simulink model "Bioreactor2_fuzzy_control"  (R2016a)
settings: Solver=VariableStepAuto  StartTime=0.0  StopTime=500  RelTol=1e-3
undefined symbols (not defined in the file or in its folder): Bioreactor2FuzzyMadani, Bioreactor2FuzzySugeno, evalfis
settings Model: Creator=Daniel  LastModifiedBy=Daniel

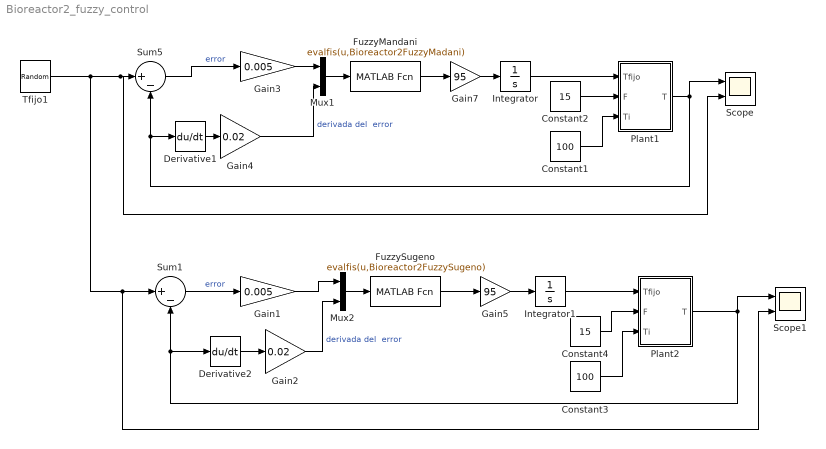
== system Bioreactor2_fuzzy_control ==
  Constant1 : Constant  Value=100
  Constant2 : Constant  Value=15
  Constant3 : Constant  Value=100
  Constant4 : Constant  Value=15
  Derivative1 : Derivative
  Derivative2 : Derivative
  FuzzyMandani : MATLABFcn  MATLABFcn=evalfis(u,Bioreactor2FuzzyMadani)  OutputDimensions=1
  FuzzySugeno : MATLABFcn  MATLABFcn=evalfis(u,Bioreactor2FuzzySugeno)  OutputDimensions=1
  Gain1 : Gain  Gain=0.005
  Gain2 : Gain  Gain=0.02
  Gain3 : Gain  Gain=0.005
  Gain4 : Gain  Gain=0.02
  Gain5 : Gain  Gain=95
  Gain7 : Gain  Gain=95
  Integrator : Integrator
  Integrator1 : Integrator
  Mux1 : Mux  Inputs=2
  Mux2 : Mux  Inputs=2
  Plant1 : Subsystem
  Plant2 : Subsystem
  Scope : Scope  NumInputPorts=2
  Scope1 : Scope  NumInputPorts=2
  Sum1 : Sum  Inputs=|+-
  Sum5 : Sum  Inputs=|+-
  Tfijo1 : UniformRandomNumber  Minimum=130  Maximum=170  SampleTime=50
  wires:
  Sum5/1 -> Gain3/1  "error"
  Gain3/1 -> Mux1/1
  Derivative1/1 -> Gain4/1
  Gain4/1 -> Mux1/2  "derivada del  error"
  Plant1/1(T) -> Scope/1, Derivative1/1, Sum5/2
  Integrator/1 -> Plant1/1(Tfijo)
  Constant2/1 -> Plant1/2(F)
  Constant1/1 -> Plant1/3(Ti)
  Mux1/1 -> FuzzyMandani/1
  FuzzyMandani/1 -> Gain7/1
  Gain7/1 -> Integrator/1
  Sum1/1 -> Gain1/1  "error"
  Gain1/1 -> Mux2/1
  Derivative2/1 -> Gain2/1
  Gain2/1 -> Mux2/2  "derivada del  error"
  Constant4/1 -> Plant2/2(F)
  Tfijo1/1 -> Scope/2, Sum5/1, Sum1/1, Scope1/2
  Constant3/1 -> Plant2/3(Ti)
  Mux2/1 -> FuzzySugeno/1
  Plant2/1(T) -> Scope1/1, Derivative2/1, Sum1/2
  FuzzySugeno/1 -> Gain5/1
  Gain5/1 -> Integrator1/1
  Integrator1/1 -> Plant2/1(Tfijo)

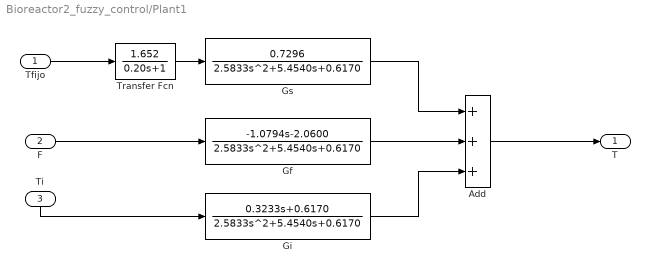
== system Bioreactor2_fuzzy_control/Plant1 ==
  Tfijo : Inport
  F : Inport  Port=2
  Ti : Inport  Port=3
  Add : Sum  Inputs=+++
  Gf : TransferFcn  Numerator=[-1.0794 -2.0600]  Denominator=[2.5833 5.4540 0.6170]
  Gi : TransferFcn  Numerator=[0.3233 0.6170]  Denominator="[2.5833 5.4540  0.6170]"
  Gs : TransferFcn  Numerator=[0.7296]  Denominator="[2.5833 5.4540  0.6170]"
  Transfer Fcn : TransferFcn  Numerator=[1.652]  Denominator=[0.20 1]
  T : Outport
  wires:
  Add/1 -> T/1
  Gi/1 -> Add/3
  Gf/1 -> Add/2
  Transfer Fcn/1 -> Gs/1
  Gs/1 -> Add/1
  Ti/1 -> Gi/1
  Tfijo/1 -> Transfer Fcn/1
  F/1 -> Gf/1

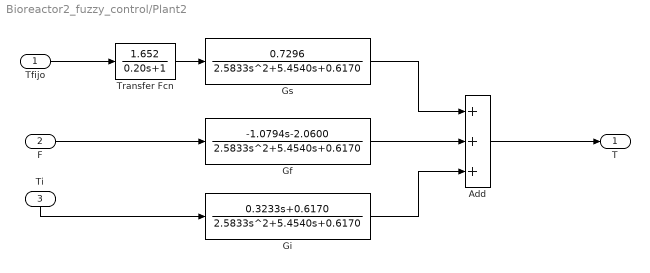
== system Bioreactor2_fuzzy_control/Plant2 ==
  Tfijo : Inport
  F : Inport  Port=2
  Ti : Inport  Port=3
  Add : Sum  Inputs=+++
  Gf : TransferFcn  Numerator=[-1.0794 -2.0600]  Denominator=[2.5833 5.4540 0.6170]
  Gi : TransferFcn  Numerator=[0.3233 0.6170]  Denominator="[2.5833 5.4540  0.6170]"
  Gs : TransferFcn  Numerator=[0.7296]  Denominator="[2.5833 5.4540  0.6170]"
  Transfer Fcn : TransferFcn  Numerator=[1.652]  Denominator=[0.20 1]
  T : Outport
  wires:
  Add/1 -> T/1
  Gi/1 -> Add/3
  Gf/1 -> Add/2
  Transfer Fcn/1 -> Gs/1
  Gs/1 -> Add/1
  Ti/1 -> Gi/1
  Tfijo/1 -> Transfer Fcn/1
  F/1 -> Gf/1
